simulink model "blikingled_28069M_launchpad"  (R2023a)
settings: Solver=FixedStepAuto  StartTime=0.0  StopTime=Inf  RelTol=1e-3
undefined symbols (not defined in the file or in its folder): Down, GPTRIP1SEL, GPTRIP2SEL, TZ1, TZ2, Up
libraries: c2802xlib x4, c2806xlib x3, c2000lib x1
settings Model: SimulationMode=external  ExtModeTrigDuration=8  Creator=citcea  LastModifiedBy=citcea
settings OptimizationCC: DefaultUnderspecifiedDataType=single  EnhancedBackFolding=on  PassReuseOutputArgsThreshold=0  MaxStackSize=1024  OptimizeBlockOrder=speed  DifferentSizesBufferReuse=on  OptimizationCustomize=off  DenormalBehavior=FlushToZero
settings DebuggingCC: ParameterTunabilityLossMsg=error
settings HardwareCC: ProdBitPerChar=16  ProdBitPerInt=16  ProdBitPerPointer=32  ProdBitPerSizeT=32  ProdBitPerPtrDiffT=32  ProdLargestAtomicInteger=Integer  ProdLargestAtomicFloat=None  ProdWordSize=16  ProdLongLongMode=on  ProdHWDeviceType=Texas Instruments->C2000
settings ModelReferenceCC: ModelReferenceNumInstancesAllowed=Single
settings SFSimCC: MATLABDynamicMemAlloc=off
settings RTWCC: Description=Embedded Coder  SystemTargetFile=ert.tlc  HardwareBoard=TI Piccolo F28069M LaunchPad  TemplateMakefile=ert_default_tmf  Toolchain=Texas Instruments Code Composer Studio (C2000)
settings CodeAppCC: ForceParamTrailComments=on  OperatorAnnotations=on
settings ERTTargetCC: CodeReplacementLibrary=TI C28x  ERTCustomFileBanners=off  SupportContinuousTime=on  SupportNonInlinedSFcns=on  RemoveResetFunc=off  ModelStepFunctionPrototypeControlCompliant=off  ExtModeTransport=4  ExtModeStaticAlloc=on  ExtModeAutomaticAllocSize=off  ExtModeStaticAllocSize=2000  ExtModeMexFile=ext_xcp  ExtModeIntrfLevel=Level2 - Open

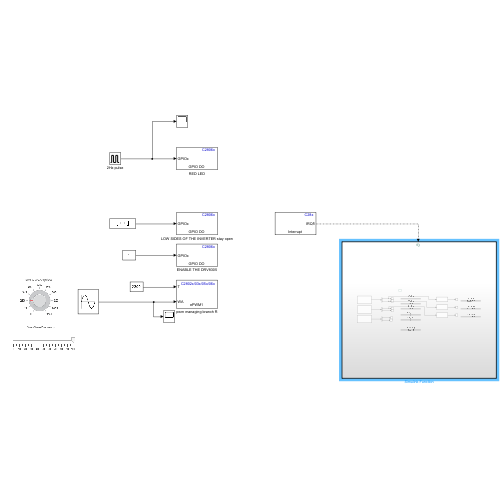
[thumbnail: Simulink's stored preview of the top-level diagram]
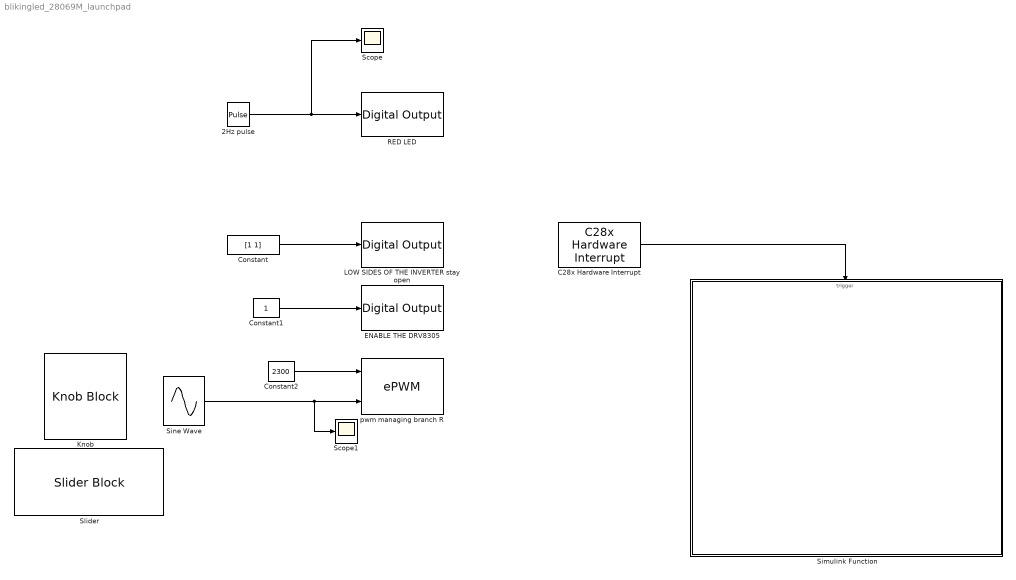
== system blikingled_28069M_launchpad ==
  2Hz pulse : DiscretePulseGenerator  PulseType=Time based  Period=0.5  PulseWidth=50
  C28x Hardware Interrupt : c2000lib/Scheduling/C28x Hardware Interrupt  irqnumbers=[1]  pienumbers=[1]  irqpriorities=[30]  irqpreempts=[1]  showinput=off  dspchiptype=C280X
  Constant : Constant  Value=[1 1]
  Constant1 : Constant
  Constant2 : Constant  Value=2300
  ENABLE THE DRV8305 : c2806xlib/Digital Output  GPIO_Number=GPIO50~GPIO55  GPIO_Bit0=off  GPIO_BIT0_Toggle=off  GPIO_Bit1=off  GPIO_BIT1_Toggle=off  GPIO_Bit2=on  GPIO_BIT2_Toggle=off  GPIO_Bit3=off  GPIO_BIT3_Toggle=off  GPIO_Bit4=off  GPIO_BIT4_Toggle=off  GPIO_Bit5=off  GPIO_BIT5_Toggle=off  GPIO_Bit6=off  GPIO_BIT6_Toggle=off  GPIO_Bit7=off  GPIO_BIT7_Toggle=off
  Knob : KnobBlock  ScaleMax=1150
  LOW SIDES OF THE INVERTER stay open : c2806xlib/Digital Output  GPIO_Number=GPIO0~GPIO7  GPIO_Bit0=off  GPIO_BIT0_Toggle=off  GPIO_Bit1=off  GPIO_BIT1_Toggle=off  GPIO_Bit2=off  GPIO_BIT2_Toggle=off  GPIO_Bit3=on  GPIO_BIT3_Toggle=off  GPIO_Bit4=off  GPIO_BIT4_Toggle=off  GPIO_Bit5=on  GPIO_BIT5_Toggle=off  GPIO_Bit6=off  GPIO_BIT6_Toggle=off  GPIO_Bit7=off  GPIO_BIT7_Toggle=off
  RED LED : c2806xlib/Digital Output  GPIO_Number=GPIO32~GPIO39  GPIO_Bit0=off  GPIO_BIT0_Toggle=off  GPIO_Bit1=off  GPIO_BIT1_Toggle=off  GPIO_Bit2=on  GPIO_BIT2_Toggle=off  GPIO_Bit3=off  GPIO_BIT3_Toggle=off  GPIO_Bit4=off  GPIO_BIT4_Toggle=off  GPIO_Bit5=off  GPIO_BIT5_Toggle=off  GPIO_Bit6=off  GPIO_BIT6_Toggle=off  GPIO_Bit7=off  GPIO_BIT7_Toggle=off
  Scope : Scope
  Scope1 : Scope
  Simulink Function : Subsystem  TreatAsAtomicUnit=on
  Sine Wave : Sin  Amplitude=227.7826404571533  Bias=2300  Frequency=100  SampleTime=0
  Slider : SliderBlock
  pwm managing branch R : c2802xlib/ePWM  PwmType=C2000  useModule=ePWM1  ePWMxLINKTBPRD=Not Linked  periodUnits=Clock cycles  timerSource=Input port  timerPeriod_clk=64000  timerPeriod_sec=0.0001  tbshadow=Counter equals to zero  countingMode=Up-Down  phaseActiveEnable=Disable  phaseDirection=Count down after sync  phaseActive=0  synchronizationEnable=off  dcaevt1Sync=off  dcbevt1Sync=off  synchronizationOption=Disable  dcbevt1SyncOut=off  dcaevt1SyncOut=off  cmpdSyncOut=off  cmpcSyncOut=off  cmpbSyncOut=off  zeroSyncOut=off  swfSyncOut=off  perSynchronizationOption=Counter equals to period (CTR=PRD)  clockPrescale=1  HSclockPrescale=1  enswap=off  ePWMxAStatus=on  ePWMxAactionLogic1=Set  ePWMxAactionLogic2=Clear  ePWMxAactionLogic3=Clear  ePWMxAactionLogic4=Set  ePWMxAactionLogic5=Do nothing  ePWMxAactionLogic6=Do nothing  ePWMxACSFenable=off  ePWMxACSFvalue=Forcing disable  ePWMxASFreload=Zero  ePWMxBStatus=off  ePWMxBactionLogic1=Set  ePWMxBactionLogic2=Clear  ePWMxBactionLogic3=Do nothing  ePWMxBactionLogic4=Do nothing  ePWMxBactionLogic5=Clear  ePWMxBactionLogic6=Set  ePWMxBCSFenable=off  ePWMxBCSFvalue=Forcing disable  ePWMxBSFreload=Zero  ePWNxBOutWay=off  ePWMxLINKCMPA=Not Linked  CMPAUnits=Clock cycles  CMPASource=Input port  CMPAValue_per=50  CMPAValue_clk=32000  enCMPAshadow=Counter equals to zero (CTR=Zero)  ePWMxLINKCMPB=Not Linked  CMPBUnits=Clock cycles  CMPBSource=Specify via dialog  CMPBValue_per=50  CMPBValue_clk=32000  enCMPBshadow=Counter equals to zero (CTR=Zero)  ePWMxLINKCMPC=Not Linked  CMPCUnits=Clock cycles  CMPCSource=Specify via dialog  CMPCValue_per=50  CMPCValue_clk=32000  enCMPCshadow=Counter equals to zero (CTR=Zero)  ePWMxLINKCMPD=Not Linked  CMPDUnits=Clock cycles  CMPDSource=Specify via dialog  CMPDValue_per=50  CMPDValue_clk=32000  enCMPDshadow=Counter equals to zero (CTR=Zero)  enableDBePWMxA=off  enableDBePWMxB=off  enhalfcycle=off  DBpolarity=Active high (AH)  DBedgeDelay=Positive  DBSource_ePWMxA=ePWMxA  DBSource_ePWMxB=ePWMxA  DBPeriodUnits=Clock cycles  DBperiodSource=Specify via dialog  REDperiod=0  FEDperiod=0  REDperiod_sec=0  FEDperiod_sec=0  LoadModeDBRED=Immediate without using shadow  LoadModeDBFED=Immediate without using shadow  adcstartModuleA=on  adcrequestEventA=First event  adcstartEventA=Counter equals to zero (CTR=Zero)  adcstartEventA_type2=Digital Compare Module A Event 1 start of conversion (DCAEVT1.soc)  adcstartModuleB=off  adcrequestEventB=First event  adcstartEventB=Counter equals to zero (CTR=Zero)  adcstartEventB_type2=Counter equals to zero (CTR=Zero)  intEn=off  intPrd=First event  intSel=Counter equals to zero (CTR=Zero)  intSel_type2=Counter equals to zero (CTR=Zero)  hrpe=off  enHRPWM=off  HRPWM_LoadMode=Counter equals to period (CTR=PRD)  HRPWM_CTLMode=Duty or Period control mode  HRPWM_EDGMode=Both edge  hrpeb=off  enHRPWMB=off  HRPWM_LoadModeB=Counter equals to zero (CTR=ZERO)  HRPWM_CTLModeB=Duty or Period control mode  HRPWM_EDGModeB=Both edge  enHRDBRED=off  enHRDBFED=off  enSFO=on  enautoconv=on  chopperEnable=off  chopperFrequency=1  chopperFirstwidth=1  chopperDuty=12.5%  tripZonesource=Specify via dialog  tzselOSHT1=off  tzselOSHT2=off  tzselOSHT3=off  tzselOSHDCAEV1=off  tzselOSHDCBEV1=off  tzselCBC1=off  tzselCBC2=off  tzselCBC3=off  tzselCBCDCAEV2=off  tzselCBCDCBEV2=off  tzselOSHT4=off  tzselOSHT5=off  tzselOSHT6=off  tzselCBC4=off  tzselCBC5=off  tzselCBC6=off  enTzOstIntr=off  enTzCbcIntr=off  enTzDCAEVT1Intr=off  enTzDCAEVT2Intr=off  enTzDCBEVT1Intr=off  enTzDCBEVT2Intr=off  ePWMxAforced=No action  ePWMxBforced=No action  DCAEVT1forced=No action  DCBEVT1forced=No action  DCAEVT2forced=No action  DCBEVT2forced=No action  dcah=Trip Zone 1 input (TZ1)  dcal=Trip Zone 1 input (TZ1)  dcbh=Trip Zone 1 input (TZ1)  dcbl=Trip Zone 1 input (TZ1)  dcah_type2=GPTRIP1SEL/(TZ1)  dcal_type2=GPTRIP2SEL/(TZ2)  dcbh_type2=GPTRIP1SEL/(TZ1)  dcbl_type2=GPTRIP2SEL/(TZ2)  gendcaevt1=Event disabled  gendcaevt2=Event disabled  gendcbevt1=Event disabled  gendcbevt2=Event disabled  dcaevt1src=DCAEVT1 with sync  dcaevt2src=DCAEVT2 with sync  dcbevt1src=DCBEVT1 with sync  dcbevt2src=DCBEVT2 with sync  pulsesel=Counter equals to zero (CTR=Zero)  blankinv=off  blankoffset=0  blankwidth=0  evsrcsel=Filtered version of DCAEVT1 (DCAEVT1FILT)  encape=off
      settings: LibrarySourceBlock=c2806xlib/ePWM
  wires:
  2Hz pulse/1 -> RED LED/1, Scope/1
  Constant/1 -> LOW SIDES OF THE INVERTER stay open/1
  Constant1/1 -> ENABLE THE DRV8305/1
  Constant2/1 -> pwm managing branch R/1
  Sine Wave/1 -> Scope1/1, pwm managing branch R/2
  C28x Hardware Interrupt/1 -> Simulink Function/Trigger

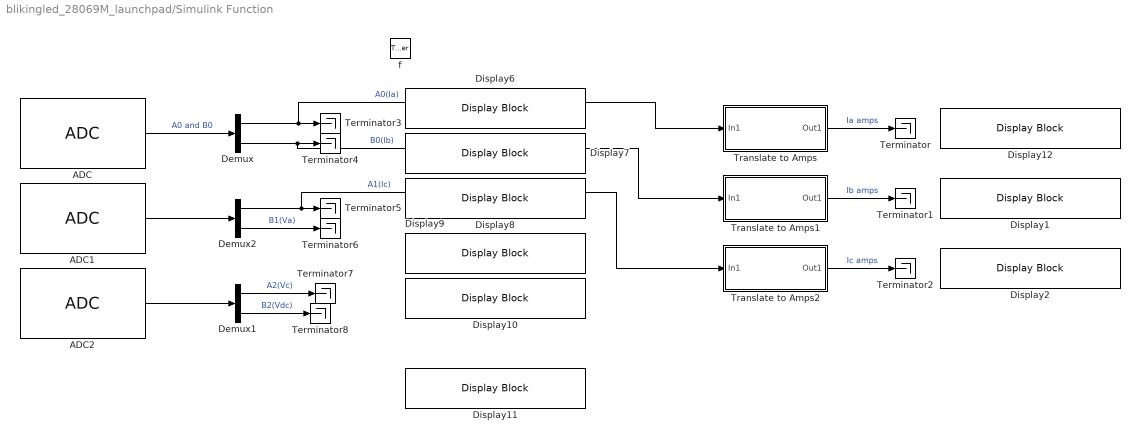
== system blikingled_28069M_launchpad/Simulink Function ==
  f : TriggerPort  TriggerType=function-call  AsynchronousFunction=on  FunctionName=f  FunctionVisibility=scoped  VariantControl=(inherit)
  ADC : c2802xlib/ADC  blkParamProc=C2000  ADCModule=1  samplingMode=Simultaneous sample mode  ADCResolution=12-bit (Single-ended input)  useSOC1=SOC0  useSOC2=SOC0_SOC1  SOCAcquisitionWindow=7  SOCTriggerSource=ePWM1_ADCSOCA  SOCInterruptTrigger=No ADCINT  Ts=-1  dType=uint16  postInterrupt=off  interruptSel=ADCINT1  ADCINTContinuous=on  endma=off  chdma=1  conv1=ADCINA0  conv2=ADCINA0 and ADCINB0  conv1_Type4=ADCIN0  conv2_Type4=ADCIN0 and ADCIN1
      settings: LibrarySourceBlock=c2806xlib/ADC
  ADC1 : c2802xlib/ADC  blkParamProc=C2000  ADCModule=1  samplingMode=Simultaneous sample mode  ADCResolution=12-bit (Single-ended input)  useSOC1=SOC1  useSOC2=SOC2_SOC3  SOCAcquisitionWindow=7  SOCTriggerSource=ePWM1_ADCSOCA  SOCInterruptTrigger=No ADCINT  Ts=-1  dType=uint16  postInterrupt=off  interruptSel=ADCINT1  ADCINTContinuous=on  endma=off  chdma=1  conv1=ADCINA1  conv2=ADCINA1 and ADCINB1  conv1_Type4=ADCIN0  conv2_Type4=ADCIN0 and ADCIN1
      settings: LibrarySourceBlock=c2806xlib/ADC
  ADC2 : c2802xlib/ADC  blkParamProc=C2000  ADCModule=1  samplingMode=Simultaneous sample mode  ADCResolution=12-bit (Single-ended input)  useSOC1=SOC2  useSOC2=SOC4_SOC5  SOCAcquisitionWindow=7  SOCTriggerSource=ePWM1_ADCSOCA  SOCInterruptTrigger=No ADCINT  Ts=-1  dType=uint16  postInterrupt=on  interruptSel=ADCINT1  ADCINTContinuous=on  endma=off  chdma=1  conv1=ADCINA2  conv2=ADCINA2 and ADCINB2  conv1_Type4=ADCIN0  conv2_Type4=ADCIN0 and ADCIN1
      settings: LibrarySourceBlock=c2806xlib/ADC
  Demux : Demux  Outputs=2
  Demux1 : Demux  Outputs=2
  Demux2 : Demux  Outputs=2
  Display{1..2,6..12} (9 alike) : DisplayBlock  Transparency=1
  Terminator{,1..8} (9 alike) : Terminator
  Translate to Amps : Subsystem  mask{Gain=1, Offset=4095/2}
      mask prompts: Gain "Introduce gain"; Offset "Introduce offset"
  Translate to Amps1 : Subsystem  mask{Gain=1, Offset=4095/2}
      mask prompts: Gain "Introduce gain"; Offset "Introduce offset"
  Translate to Amps2 : Subsystem  mask{Gain=1, Offset=4095/2}
      mask prompts: Gain "Introduce gain"; Offset "Introduce offset"
  wires:
  Demux2/2 -> Terminator6/1  "B1(Va)"
  Demux2/1 -> Translate to Amps2/1(In1), Terminator5/1  "A1(Ic)"
  Demux1/2 -> Terminator8/1  "B2(Vdc)"
  ADC/1 -> Demux/1  "A0 and B0"
  Demux/1 -> Translate to Amps/1(In1), Terminator3/1  "A0(Ia)"
  Demux/2 -> Translate to Amps1/1(In1), Terminator4/1  "B0(Ib)"
  Demux1/1 -> Terminator7/1  "A2(Vc)"
  ADC2/1 -> Demux1/1
  ADC1/1 -> Demux2/1
  Translate to Amps/1(Out1) -> Terminator/1  "Ia amps"
  Translate to Amps1/1(Out1) -> Terminator1/1  "Ib amps"
  Translate to Amps2/1(Out1) -> Terminator2/1  "Ic amps"

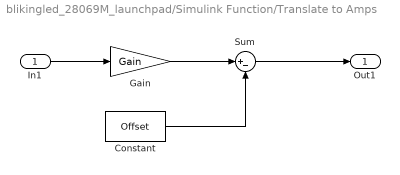
== system blikingled_28069M_launchpad/Simulink Function/Translate to Amps ==
  In1 : Inport
  Constant : Constant  Value=Offset
  Gain : Gain  Gain=Gain
  Sum : Sum  Inputs=|+-
  Out1 : Outport
  wires:
  In1/1 -> Gain/1
  Sum/1 -> Out1/1
  Constant/1 -> Sum/2
  Gain/1 -> Sum/1

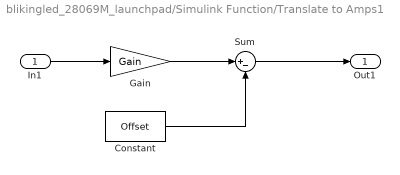
== system blikingled_28069M_launchpad/Simulink Function/Translate to Amps1 ==
  In1 : Inport
  Constant : Constant  Value=Offset
  Gain : Gain  Gain=Gain
  Sum : Sum  Inputs=|+-
  Out1 : Outport
  wires:
  In1/1 -> Gain/1
  Sum/1 -> Out1/1
  Constant/1 -> Sum/2
  Gain/1 -> Sum/1

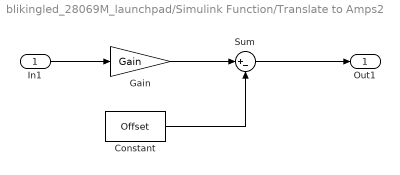
== system blikingled_28069M_launchpad/Simulink Function/Translate to Amps2 ==
  In1 : Inport
  Constant : Constant  Value=Offset
  Gain : Gain  Gain=Gain
  Sum : Sum  Inputs=|+-
  Out1 : Outport
  wires:
  In1/1 -> Gain/1
  Sum/1 -> Out1/1
  Constant/1 -> Sum/2
  Gain/1 -> Sum/1
